simulink model "SixDOF_v2_1c"  (R2019b)
settings: Solver=ode4  StartTime=0  StopTime=200  FixedStep=0.01  RelTol=1e-3
libraries: aerolibconvert2 x11, dspsrcs4 x4, simulink x2
settings Model: SimulationMode=accelerator  Creator=Jared  LastModifiedBy=j90xb
settings SolverCC: AlgebraicLoopSolver=LineSearch
settings DataIOCC: SaveFormat=Array  ReturnWorkspaceOutputs=off
settings DebuggingCC: ArithmeticOperatorsInVariantConditions=warning
settings SFSimCC: SimUseLocalCustomCode=off  CustomCodeUndefinedFunction=UseInterfaceOnly
settings RTWCC: RTWUseLocalCustomCode=off

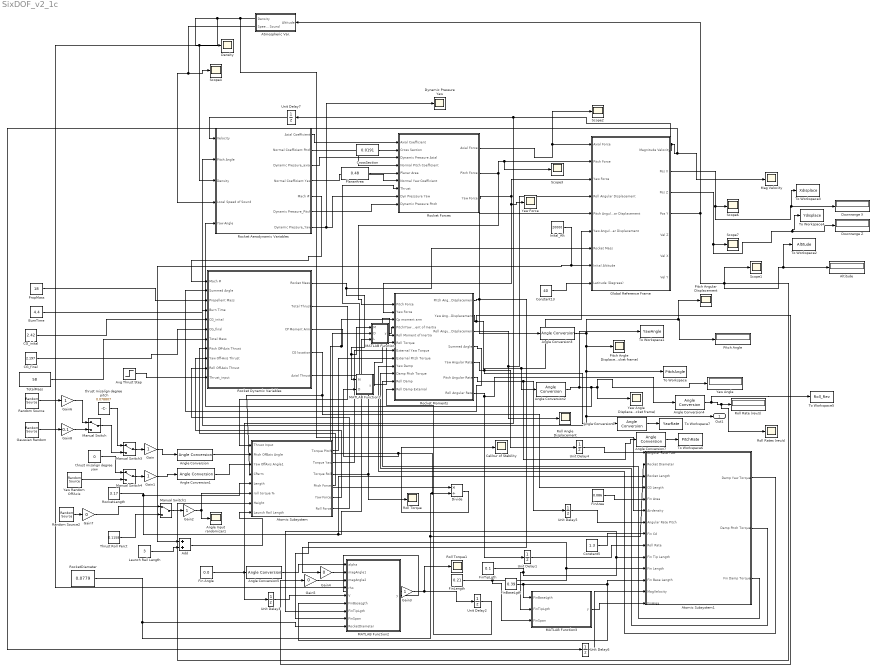
== system SixDOF_v2_1c ==
  Add : Sum
  Altitude : Display
  Angle Conversion : aerolibconvert2/Angle Conversion  IU=deg  OU=rad
  Angle Conversion1 : aerolibconvert2/Angle Conversion  IU=deg  OU=rad
  Angle Conversion{2..3,6..7} (4 alike) : aerolibconvert2/Angle Conversion  IU=rad  OU=deg
  Angle Conversion4 : aerolibconvert2/Angle Conversion  IU=rad  OU=rev
  Angle Conversion5 : aerolibconvert2/Angle Conversion  IU=deg  OU=rad
  Angle Input randomizer1 : Scope
  Atmospheric Var. : Subsystem  TreatAsAtomicUnit=on
  Atomic Subsystem : Subsystem  TreatAsAtomicUnit=on
  Atomic Subsystem1 : Subsystem  TreatAsAtomicUnit=on
  Avg Thrust Step : Step  Time=4.4  Before=8000  After=0
  BurnTime : Constant  Value=4.4
  CG_final : Constant  Value=2.197
  CG_inital : Constant  Value=2.42
  Calibur of Stability : Scope
  Constant13 : Constant  Value=40
  Constant5 : Constant  Value=1.3
  CrossSection : Constant  Value=0.0191
  Density : Scope
  Divide : Product  Inputs=*/
  Downrange X : Display
  Downrange Z : Display
  Dynamic Pressure Yaw : Scope
  Fin Angle : Constant  Value=0.0
  FinArea : Constant  Value=0.086
  FinBaseLgth : Constant  Value=0.39
  FinLength : Constant  Value=0.21
  FinTipLgth : Constant  Value=0.1
  Gain{,1..3,6} (5 alike) : Gain
  Gain4 : Gain  Gain=0
  Gain5 : Gain  Gain=0
  Gain7 : Gain  Gain=0
  Gain8 : Gain  Gain=0.1
  Gaussian Random : dspsrcs4/Random Source  SrcType=Gaussian  NormMethod=Ziggurat  CltLength=12  MinVal=-0.2  MaxVal=0.2  MeanVal=0  VarVal=1  RepMode=Not repeatable  rawSeed=1  IsInherit=off  SampMode=Discrete  SampTime=1  SampFrame=1  DataType=Double  OutComplex=Real  OutputFrames=off
  Global Reference Frame : Subsystem  TreatAsAtomicUnit=on
  Inital_Alt : Constant  Value=20000
  Launch Rail Length : Constant  Value=3
  MATLAB Function : MATLAB Function  TreatAsAtomicUnit=on
  MATLAB Function1 : MATLAB Function  TreatAsAtomicUnit=on
  MATLAB Function2 : MATLAB Function  TreatAsAtomicUnit=on
  MATLAB Function3 : MATLAB Function  TreatAsAtomicUnit=on
  Mag Velocity : Scope
  Manual Switch{,1,3..4} (4 alike) : ManualSwitch
  Pitch Angle : Display
  Pitch Angle Displacement (rocket frame) : Scope
  Pitch Angular Displacement : Scope
  PlanarArea : Constant  Value=0.48
  PropMass : Constant  Value=18
  Random Source : dspsrcs4/Random Source  SrcType=Uniform  NormMethod=Ziggurat  CltLength=12  MinVal=-0.2  MaxVal=0.2  MeanVal=0  VarVal=1  RepMode=Not repeatable  rawSeed=1  IsInherit=off  SampMode=Discrete  SampTime=1000  SampFrame=1  DataType=Double  OutComplex=Real  OutputFrames=off
  Random Source2 : dspsrcs4/Random Source  SrcType=Uniform  NormMethod=Ziggurat  CltLength=12  MinVal=-0.001  MaxVal=0.001  MeanVal=0  VarVal=1  RepMode=Not repeatable  rawSeed=1  IsInherit=off  SampMode=Discrete  SampTime=0.5  SampFrame=1  DataType=Double  OutComplex=Real  OutputFrames=off
  Rocket Aerodynamic Variables : Subsystem  TreatAsAtomicUnit=on
  "Rocket Dynamic Variables " : Subsystem  TreatAsAtomicUnit=on
  Rocket Forces : Subsystem  TreatAsAtomicUnit=on
  Rocket Moments : Subsystem  TreatAsAtomicUnit=on
  RocketDiameter : Constant  Value=0.0779
  RocketLength : Constant  Value=3.17
  Roll Angle Displacement : Scope
  Roll Rate (rev/s) : Display
  Roll Rates (rev/s) : Scope
  Roll Torque : Scope
  Roll Torque1 : Scope
  Scope{1..4,6..7} (6 alike) : Scope
  Thrust Roll Perct : Constant  Value=0.1158
  To Workspace : ToWorkspace  VariableName=PitchAngle  SampleTime=-1
  To Workspace1 : ToWorkspace  VariableName=YawAngle  SampleTime=-1
  To Workspace2 : ToWorkspace  VariableName=Altitude  SampleTime=-1
  To Workspace3 : ToWorkspace  VariableName=Xdisplace  SampleTime=-1
  To Workspace4 : ToWorkspace  VariableName=Ydisplace  SampleTime=-1
  To Workspace5 : ToWorkspace  VariableName=Roll_Rev  SampleTime=-1
  To Workspace6 : ToWorkspace  VariableName=PitchRate  SampleTime=-1
  To Workspace7 : ToWorkspace  VariableName=YawRate  SampleTime=-1
  TotalMass : Constant  Value=58
  Unit Delay{1..7} (7 alike) : UnitDelay  SampleTime=-1  HasFrameUpgradeWarning=on
  Yaw Angle : Display
  Yaw Angle Displacement (rocket frame) : Scope
  Yaw Force : Scope
  Yaw Random OffAxis : dspsrcs4/Random Source  SrcType=Uniform  NormMethod=Ziggurat  CltLength=12  MinVal=-0.02  MaxVal=0.02  MeanVal=0  VarVal=1  RepMode=Not repeatable  rawSeed=1  IsInherit=off  SampMode=Discrete  SampTime=1000  SampFrame=1  DataType=Double  OutComplex=Real  OutputFrames=off
  thrust misalign degree pitch : Constant  Value=0.078807
  thrust misalign degree yaw : Constant  Value=0
  Out1 : Outport  VectorParamsAs1DForOutWhenUnconnected=off
  wires:
  Rocket Forces/1(Axial Force) -> Scope2/1, Global Reference Frame/1(Axial Force)
  Rocket Moments/1(Pitch Angular Displacement) -> Gain4/1, Angle Conversion3/1, Global Reference Frame/5(Pitch Angular Displacement)
  Global Reference Frame/1(Magnitude Velocity) -> Unit Delay3/1, Unit Delay7/1, Unit Delay6/1, Mag Velocity/1
  Global Reference Frame/4(Pos Y) -> Atmospheric Var./1(Altitude), Atomic Subsystem/7(Height), To Workspace2/1, Altitude/1, Scope1/1
  "Rocket Dynamic Variables "/3(CP Moment Arm) -> Divide/1, Rocket Moments/3(Cp moment arm)
  PropMass/1 -> "Rocket Dynamic Variables "/3(Propellent Mass)
  BurnTime/1 -> "Rocket Dynamic Variables "/4(Burn Time)
  CG_inital/1 -> "Rocket Dynamic Variables "/5(CG_inital)
  CG_final/1 -> "Rocket Dynamic Variables "/6(CG_final)
  TotalMass/1 -> "Rocket Dynamic Variables "/7(Total Mass)
  MATLAB Function/1(y) -> Rocket Moments/4(Pitch/Yaw Moment of Inertia)
  CrossSection/1 -> Rocket Forces/2(Cross Section)
  PlanarArea/1 -> Rocket Forces/5(Planar Area)
  Inital_Alt/1 -> Add/1, Global Reference Frame/8(Inital Altitude)
  Atmospheric Var./2(Speed of Sound) -> Scope4/1, Rocket Aerodynamic Variables/4(Local Speed of Sound)
  Global Reference Frame/2(Pos X) -> To Workspace3/1, Downrange X/1, Scope6/1
  Global Reference Frame/3(Pos Z) -> To Workspace4/1, Downrange Z/1, Scope7/1
  Atomic Subsystem/1(Torque Pitch) -> Rocket Moments/8(External Pitch Torque)
  Atomic Subsystem/2(Torque Yaw) -> Rocket Moments/7(External Yaw Torque)
  Angle Conversion/1 -> Atomic Subsystem/2(Pitch OffAxis Angle)
  Angle Conversion1/1 -> Atomic Subsystem/3(Yaw OffAxis Angle1)
  RocketLength/1 -> Atomic Subsystem1/3(Rocket Length), MATLAB Function/3(L), Atomic Subsystem/5(Length)
  Divide/1 -> Calibur of Stability/1
  Atomic Subsystem/3(Torque Roll) -> Roll Torque/1, Rocket Moments/6(Roll Torque)
  MATLAB Function1/1(y) -> Rocket Moments/5(Roll Moment of Inertia)
  Gain/1 -> Angle Conversion/1
  Gain1/1 -> Angle Conversion1/1
  Gain2/1 -> Atomic Subsystem/6(roll torque %), Angle Input randomizer1/1
  RocketDiameter/1 -> MATLAB Function2/9(RocketDiameter), Atomic Subsystem1/2(Rocket Diameter), MATLAB Function1/2(D), MATLAB Function/2(D), Divide/2
  "Rocket Dynamic Variables "/4(CG location) -> Atomic Subsystem1/4(CG Length), Atomic Subsystem/4(CParm)
  "Rocket Dynamic Variables "/1(Rocket Mass) -> MATLAB Function/1(M), MATLAB Function1/1(M), Global Reference Frame/7(Rocket Mass)
  Rocket Forces/3(Yaw Force) -> Rocket Moments/2(Yaw Force), Yaw Force/1, Global Reference Frame/3(Yaw Force)
  Rocket Moments/3(Roll Angular Displacement) -> Roll Angle Displacement/1, Global Reference Frame/4(Roll Angular Displacement)
  "Rocket Dynamic Variables "/5(Axial Thrust) -> Rocket Forces/7(Thrust)
  Rocket Aerodynamic Variables/5(Mach #) -> "Rocket Dynamic Variables "/1("Mach # ")
  Rocket Aerodynamic Variables/1(" Axial Coefficient") -> Rocket Forces/1(Axial Coefficient)
  Rocket Aerodynamic Variables/3(Dynamic Pressure_axial) -> Rocket Forces/3(Dynamic Pressure Axial)
  Rocket Aerodynamic Variables/2(" Normal Coefficient Pitch") -> Rocket Forces/4(Normal Pitch Coefficient)
  Rocket Aerodynamic Variables/4(" Normal Coefficient Yaw") -> Rocket Forces/6(Normal Yaw Coefficient)
  "Rocket Dynamic Variables "/2(Total Thrust) -> Atomic Subsystem/1(Thrust Input)
  Atmospheric Var./1(Density) -> Atomic Subsystem1/6(Airdensity), MATLAB Function2/4(rho), Density/1, Rocket Aerodynamic Variables/3(Density)
  Rocket Moments/4(Summed Angle) -> "Rocket Dynamic Variables "/2(Summed Angle)
  Atomic Subsystem/4(Pitch Force) -> "Rocket Dynamic Variables "/8(Pitch Off-Axis Thrust)
  Atomic Subsystem/5(Yaw Force) -> "Rocket Dynamic Variables "/9(Yaw Off-Axis Thrust)
  Atomic Subsystem/6(Roll Force) -> "Rocket Dynamic Variables "/10(Roll Off-Axis Thrust)
  Rocket Aerodynamic Variables/6(Dynamic Pressure_Pitch) -> Rocket Forces/9(Dynamic Pressure Pitch)
  Rocket Aerodynamic Variables/7(Dynamic Pressure_Yaw) -> Dynamic Pressure Yaw/1, Rocket Forces/8(Dyn Presssure Yaw)
  Unit Delay7/1 -> Rocket Aerodynamic Variables/1(Velocity)
  Rocket Moments/2(Yaw Angular Displacement) -> Gain5/1, Global Reference Frame/6(Yaw Angular Displacement), Angle Conversion2/1
  Rocket Moments/5(Yaw Angular Rate) -> Angle Conversion6/1, Unit Delay4/1
  FinArea/1 -> Atomic Subsystem1/5(Fin Area)
  Atomic Subsystem1/1(Damp Yaw Torque) -> Rocket Moments/9(Yaw Damp)
  Unit Delay4/1 -> Atomic Subsystem1/1(Angular Rate Yaw)
  Angle Conversion2/1 -> To Workspace1/1, Rocket Aerodynamic Variables/5(Yaw Angle), Yaw Angle/1, Yaw Angle Displacement (rocket frame)/1
  Atomic Subsystem1/2(Damp Pitch Torque) -> Rocket Moments/10(Damp Pitch Torque)
  Rocket Moments/6(Pitch Angular Rate) -> Angle Conversion7/1, Unit Delay5/1
  Unit Delay5/1 -> Atomic Subsystem1/7(Angular Rate Pitch)
  Gaussian Random/1 -> Gain8/1
  Random Source/1 -> Gain6/1
  Manual Switch1/1 -> Gain2/1
  Random Source2/1 -> Gain7/1
  Thrust Roll Perct/1 -> Manual Switch1/2
  Constant13/1 -> Global Reference Frame/9(Latitude (Degrees))
  Launch Rail Length/1 -> Add/2
  Add/1 -> Atomic Subsystem/8(Launch Rail Length)
  Angle Conversion3/1 -> Rocket Aerodynamic Variables/2(Pitch Angle), Out1/1, To Workspace/1, Pitch Angle Displacement (rocket frame)/1, Pitch Angle/1, Pitch Angular Displacement/1
  Atomic Subsystem1/3(Fin Damp Torque) -> Rocket Moments/11(Roll Damp)
  Rocket Moments/7(Roll Angular Rate) -> Angle Conversion4/1, Unit Delay1/1
  Constant5/1 -> Atomic Subsystem1/8(Fin Cd)
  FinTipLgth/1 -> MATLAB Function3/2(FinTipLgth), Atomic Subsystem1/10(Fin Tip Length), MATLAB Function2/7(FinTipLgth)
  FinLength/1 -> MATLAB Function3/3(FinSpan), MATLAB Function2/8(FinSpan), Atomic Subsystem1/11(Fin Length)
  FinBaseLgth/1 -> MATLAB Function3/1(FinBaseLgth), MATLAB Function2/6(FinBaseLgth), Atomic Subsystem1/12(Fin Base Length)
  Unit Delay1/1 -> Atomic Subsystem1/9(Roll Rate)
  MATLAB Function2/1(y) -> Gain3/1
  Angle Conversion5/1 -> MATLAB Function2/1(alpha)
  Fin Angle/1 -> Angle Conversion5/1
  Unit Delay2/1 -> Rocket Moments/12(Roll Damp External)
  Unit Delay3/1 -> MATLAB Function2/5(V)
  MATLAB Function3/1(y) -> Atomic Subsystem1/14(FinArea)
  Unit Delay6/1 -> Atomic Subsystem1/13(MagVelocity)
  Angle Conversion4/1 -> To Workspace5/1, Roll Rates (rev/s)/1, Roll Rate (rev/s)/1
  Gain3/1 -> Roll Torque1/1, Unit Delay2/1
  Rocket Forces/2(Pitch Force) -> Rocket Moments/1(Pitch Force), Scope3/1, Global Reference Frame/2(Pitch Force)
  Angle Conversion7/1 -> To Workspace6/1
  Angle Conversion6/1 -> To Workspace7/1
  Gain4/1 -> MATLAB Function2/2(magAngle1)
  Gain5/1 -> MATLAB Function2/3(magAngle2)
  Gain7/1 -> Manual Switch1/1
  Gain6/1 -> Manual Switch/1
  Gain8/1 -> Manual Switch/2
  Manual Switch3/1 -> Gain/1
  Manual Switch4/1 -> Gain1/1
  Yaw Random OffAxis/1 -> Manual Switch4/2
  Manual Switch/1 -> Manual Switch3/2
  thrust misalign degree pitch/1 -> Manual Switch3/1
  thrust misalign degree yaw/1 -> Manual Switch4/1
  Avg Thrust Step/1 -> "Rocket Dynamic Variables "/11(Thrust_input)

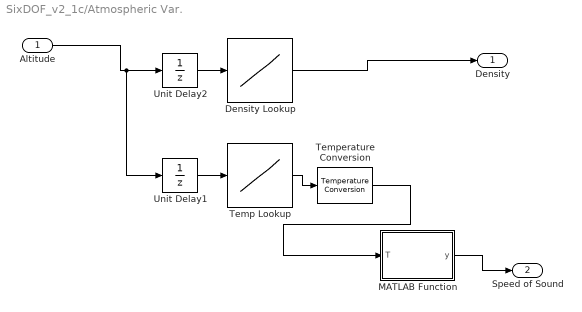
== system SixDOF_v2_1c/Atmospheric Var. ==
  Altitude : Inport
  Density Lookup : Lookup_n-D  NumberOfTableDimensions=1  BreakpointsForDimension1=[0,1000,2000,3000,4000,5000,6000,7000,8000,9000,10000,15000,20000,25000,30000,40000,50000,60000,70000,80000,120000]  Table=[1.347,1.225,1.112,1.007,0.9093,0.8194,0.7364,0.6601,0.59,0.4671,0.4135,0.1948,0.0889,0.04,0.0184,0.003996,0.001027,0.0003097,8.283e-05,0.00001846,1e-07]  InterpMethod=Cubic spline  InternalRulePriority=Speed  RndMeth=Simplest  InputSameDT=on
  MATLAB Function : MATLAB Function  TreatAsAtomicUnit=on
  Temp Lookup : Lookup_n-D  NumberOfTableDimensions=1  BreakpointsForDimension1=[0,1000,2000,3000,4000,5000,6000,7000,8000,9000,10000,15000,20000,25000,30000,40000,50000,60000,70000,80000,120000]  Table=[21.50,8.5,2,-4.49,-10.98,-17.47,-23.96,-30.45,-36.95,-43.42,-49.90,-56.50,-56.50,-51.60,-46.64,-22.80,-2.5,-26.13,-53.57,-74.51,-80]  InternalRulePriority=Speed  RndMeth=Simplest  InputSameDT=on
  Temperature Conversion : aerolibconvert2/Temperature Conversion  IU=C  OU=K
      settings: SourceProductName=Aerospace Blockset  SourceProductBaseCode=AE
  Unit Delay1 : UnitDelay  SampleTime=-1  HasFrameUpgradeWarning=on
  Unit Delay2 : UnitDelay  SampleTime=-1  HasFrameUpgradeWarning=on
  Density : Outport  VectorParamsAs1DForOutWhenUnconnected=off
  Speed of Sound : Outport  Port=2  VectorParamsAs1DForOutWhenUnconnected=off
  wires:
  Altitude/1 -> Unit Delay2/1, Unit Delay1/1
  Temp Lookup/1 -> Temperature Conversion/1
  MATLAB Function/1(y) -> Speed of Sound/1
  Temperature Conversion/1 -> MATLAB Function/1(T)
  Density Lookup/1 -> Density/1
  Unit Delay1/1 -> Temp Lookup/1
  Unit Delay2/1 -> Density Lookup/1

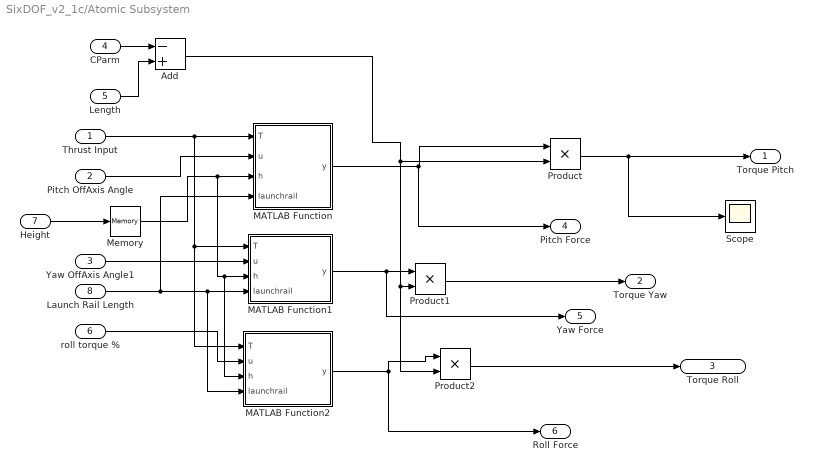
== system SixDOF_v2_1c/Atomic Subsystem ==
  Thrust Input : Inport
  Pitch OffAxis Angle : Inport  Port=2
  Yaw OffAxis Angle1 : Inport  Port=3
  CParm : Inport  Port=4
  Length : Inport  Port=5
  roll torque % : Inport  Port=6
  Height : Inport  Port=7
  Launch Rail Length : Inport  Port=8
  Add : Sum  Inputs=-+
  MATLAB Function : MATLAB Function  TreatAsAtomicUnit=on
  MATLAB Function1 : MATLAB Function  TreatAsAtomicUnit=on
  MATLAB Function2 : MATLAB Function  TreatAsAtomicUnit=on
  Memory : Memory
  Product : Product
  Product1 : Product
  Product2 : Product
  Scope : Scope
  Torque Pitch : Outport  VectorParamsAs1DForOutWhenUnconnected=off
  Torque Yaw : Outport  Port=2  VectorParamsAs1DForOutWhenUnconnected=off
  Torque Roll : Outport  Port=3  VectorParamsAs1DForOutWhenUnconnected=off
  Pitch Force : Outport  Port=4  VectorParamsAs1DForOutWhenUnconnected=off
  Yaw Force : Outport  Port=5  VectorParamsAs1DForOutWhenUnconnected=off
  Roll Force : Outport  Port=6  VectorParamsAs1DForOutWhenUnconnected=off
  wires:
  CParm/1 -> Add/1
  Length/1 -> Add/2
  MATLAB Function1/1(y) -> Yaw Force/1, Product1/1
  Product1/1 -> Torque Yaw/1
  Product2/1 -> Torque Roll/1
  MATLAB Function2/1(y) -> Product2/1, Roll Force/1
  Product/1 -> Torque Pitch/1, Scope/1
  MATLAB Function/1(y) -> Pitch Force/1, Product/1
  Add/1 -> Product2/2, Product1/2, Product/2
  Thrust Input/1 -> MATLAB Function2/1(T), MATLAB Function1/1(T), MATLAB Function/1(T)
  Pitch OffAxis Angle/1 -> MATLAB Function/2(u)
  roll torque %/1 -> MATLAB Function2/2(u)
  Yaw OffAxis Angle1/1 -> MATLAB Function1/2(u)
  Height/1 -> Memory/1
  Launch Rail Length/1 -> MATLAB Function/4(launchrail), MATLAB Function2/4(launchrail), MATLAB Function1/4(launchrail)
  Memory/1 -> MATLAB Function2/3(h), MATLAB Function1/3(h), MATLAB Function/3(h)

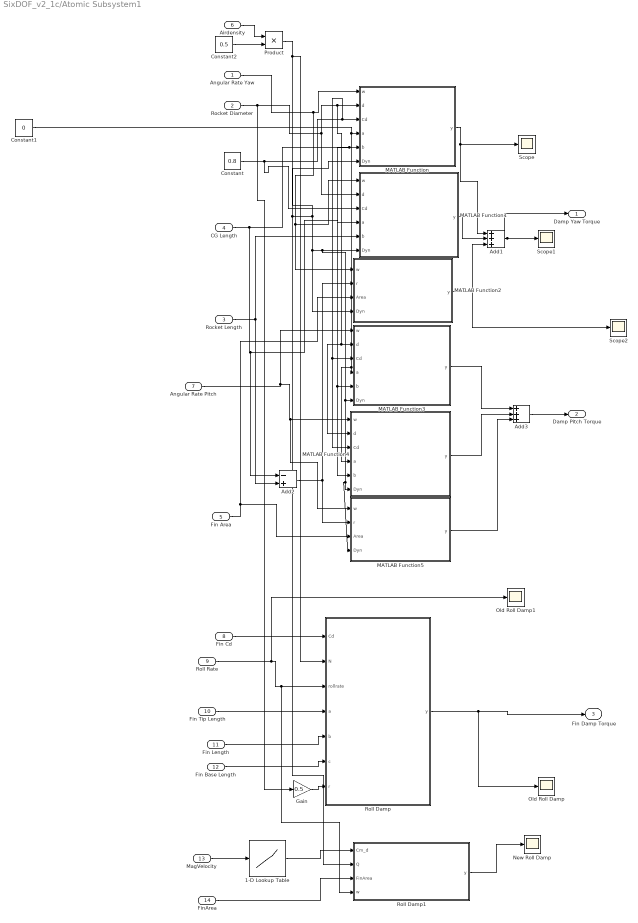
== system SixDOF_v2_1c/Atomic Subsystem1 ==
  Angular Rate Yaw : Inport
  Rocket Diameter : Inport  Port=2
  Rocket Length : Inport  Port=3
  CG Length : Inport  Port=4
  Fin Area : Inport  Port=5
  Airdensity : Inport  Port=6
  Angular Rate Pitch : Inport  Port=7
  Fin Cd : Inport  Port=8
  Roll Rate : Inport  Port=9
  Fin Tip Length : Inport  Port=10
  Fin Length : Inport  Port=11
  Fin Base Length : Inport  Port=12
  MagVelocity : Inport  Port=13
  FinArea : Inport  Port=14
  1-D Lookup Table : Lookup_n-D  NumberOfTableDimensions=1  BreakpointsForDimension1=[0,0.1,0.5,1,2,3,4,5]  Table=[2,0.65,0.61,0.75,0.25,0.2,0.18,0.17]  InternalRulePriority=Speed  RndMeth=Simplest  InputSameDT=on
  Add1 : Sum  Inputs=+++
  Add2 : Sum  Inputs=-+
  Add3 : Sum  Inputs=+++
  Constant : Constant  Value=0.8
  Constant1 : Constant  Value=0
  Constant2 : Constant  Value=0.5
  Gain : Gain  Gain=0.5
  MATLAB Function : MATLAB Function  TreatAsAtomicUnit=on
  MATLAB Function1 : MATLAB Function  TreatAsAtomicUnit=on
  MATLAB Function2 : MATLAB Function  TreatAsAtomicUnit=on
  MATLAB Function3 : MATLAB Function  TreatAsAtomicUnit=on
  MATLAB Function4 : MATLAB Function  TreatAsAtomicUnit=on
  MATLAB Function5 : MATLAB Function  TreatAsAtomicUnit=on
  New Roll Damp : Scope
  Old Roll Damp : Scope
  Old Roll Damp1 : Scope
  Product : Product
  Roll Damp : MATLAB Function  TreatAsAtomicUnit=on
  Roll Damp1 : MATLAB Function  TreatAsAtomicUnit=on
  Scope : Scope
  Scope1 : Scope
  Scope2 : Scope
  Damp Yaw Torque : Outport  VectorParamsAs1DForOutWhenUnconnected=off
  Damp Pitch Torque : Outport  Port=2  VectorParamsAs1DForOutWhenUnconnected=off
  Fin Damp Torque : Outport  Port=3  VectorParamsAs1DForOutWhenUnconnected=off
  wires:
  Angular Rate Yaw/1 -> MATLAB Function2/1(w), MATLAB Function1/1(w), MATLAB Function/1(w)
  Constant/1 -> MATLAB Function4/3(Cd), MATLAB Function3/3(Cd), MATLAB Function/3(Cd), MATLAB Function1/3(Cd)
  Constant1/1 -> MATLAB Function4/4(a), MATLAB Function3/4(a), MATLAB Function/4(a)
  MATLAB Function/1(y) -> Add1/1, Scope/1
  CG Length/1 -> Add2/1, MATLAB Function1/4(a), MATLAB Function4/5(b), MATLAB Function3/5(b), MATLAB Function/5(b)
  Rocket Length/1 -> Add2/2, MATLAB Function1/5(b)
  MATLAB Function1/1(y) -> Add1/2
  Add1/1 -> Damp Yaw Torque/1, Scope1/1
  Airdensity/1 -> Product/1
  Constant2/1 -> Product/2
  Product/1 -> Roll Damp/2(N), Roll Damp1/2(Q), MATLAB Function2/4(Dyn), MATLAB Function5/4(Dyn), MATLAB Function4/6(Dyn), MATLAB Function3/6(Dyn), MATLAB Function1/6(Dyn), MATLAB Function/6(Dyn)
  Add2/1 -> MATLAB Function2/2(r), MATLAB Function5/2(r)
  Fin Area/1 -> MATLAB Function5/3(Area), MATLAB Function2/3(Area)
  MATLAB Function2/1(y) -> Add1/3, Scope2/1
  Angular Rate Pitch/1 -> MATLAB Function5/1(w), MATLAB Function4/1(w), MATLAB Function3/1(w)
  MATLAB Function3/1(y) -> Add3/1
  MATLAB Function4/1(y) -> Add3/2
  MATLAB Function5/1(y) -> Add3/3
  Add3/1 -> Damp Pitch Torque/1
  Roll Rate/1 -> Old Roll Damp1/1, Roll Damp1/4(w), Roll Damp/3(rollrate)
  Fin Tip Length/1 -> Roll Damp/4(a)
  Gain/1 -> Roll Damp/7(r)
  Fin Base Length/1 -> Roll Damp/6(c)
  Fin Cd/1 -> Roll Damp/1(Cd)
  Fin Length/1 -> Roll Damp/5(b)
  Rocket Diameter/1 -> Gain/1, MATLAB Function1/2(d), MATLAB Function4/2(d), MATLAB Function3/2(d), MATLAB Function/2(d)
  MagVelocity/1 -> 1-D Lookup Table/1
  1-D Lookup Table/1 -> Roll Damp1/1(Cm_d)
  FinArea/1 -> Roll Damp1/3(FinArea)
  Roll Damp1/1(y) -> New Roll Damp/1
  Roll Damp/1(y) -> Old Roll Damp/1, Fin Damp Torque/1

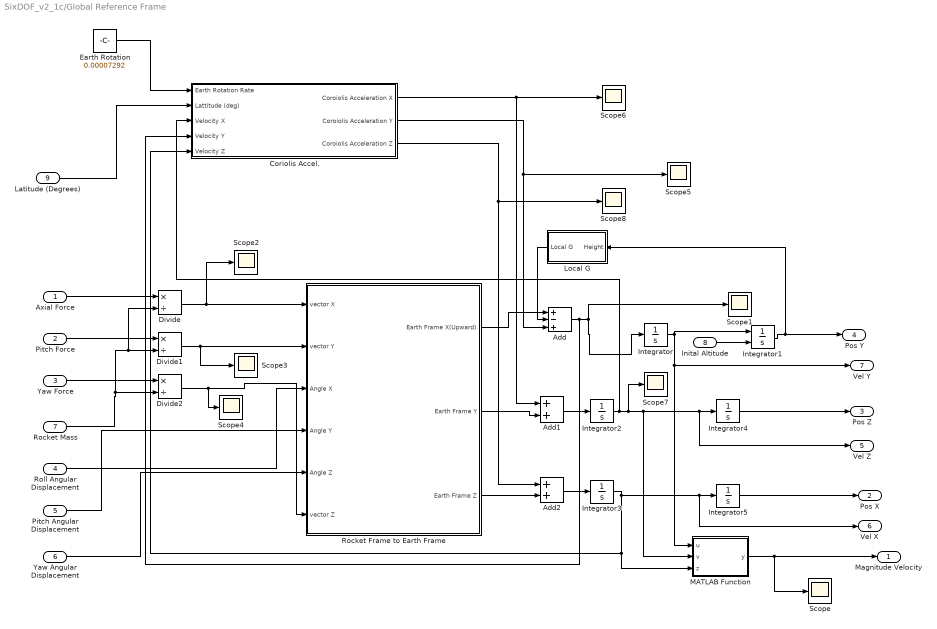
== system SixDOF_v2_1c/Global Reference Frame ==
  Axial Force : Inport
  Pitch Force : Inport  Port=2
  Yaw Force : Inport  Port=3
  Roll Angular Displacement : Inport  Port=4
  Pitch Angular Displacement : Inport  Port=5
  Yaw Angular Displacement : Inport  Port=6
  Rocket Mass : Inport  Port=7
  Inital Altitude : Inport  Port=8
  Latitude (Degrees) : Inport  Port=9
  Add : Sum  Inputs=+-+
  Add1 : Sum
  Add2 : Sum
  Coriolis Accel. : Subsystem
  Divide : Product  Inputs=*/
  Divide1 : Product  Inputs=*/
  Divide2 : Product  Inputs=*/
  Earth Rotation : Constant  Value=0.00007292
  Integrator{,2..5} (5 alike) : Integrator
  Integrator1 : Integrator  InitialConditionSource=external
  Local G : Subsystem
  MATLAB Function : MATLAB Function  TreatAsAtomicUnit=on
  Rocket Frame to Earth Frame : Subsystem
  Scope{,1..8} (9 alike) : Scope
  Magnitude Velocity : Outport  VectorParamsAs1DForOutWhenUnconnected=off
  Pos X : Outport  Port=2  VectorParamsAs1DForOutWhenUnconnected=off
  Pos Z : Outport  Port=3  VectorParamsAs1DForOutWhenUnconnected=off
  Pos Y : Outport  Port=4  VectorParamsAs1DForOutWhenUnconnected=off
  Vel Z : Outport  Port=5  VectorParamsAs1DForOutWhenUnconnected=off
  Vel X : Outport  Port=6  VectorParamsAs1DForOutWhenUnconnected=off
  "Vel Y " : Outport  Port=7  VectorParamsAs1DForOutWhenUnconnected=off
  wires:
  Divide/1 -> Rocket Frame to Earth Frame/1(vector X), Scope2/1
  Divide1/1 -> Rocket Frame to Earth Frame/2(vector Y), Scope3/1
  Divide2/1 -> Rocket Frame to Earth Frame/6(vector Z), Scope4/1
  Local G/1(Local G) -> Add/2
  Add/1 -> Coriolis Accel./4(Velocity Y), Integrator/1, Scope1/1
  Integrator3/1 -> Coriolis Accel./5(Velocity Z), MATLAB Function/3(z), Vel X/1, Integrator5/1
  Integrator5/1 -> Pos X/1
  Integrator4/1 -> Pos Z/1
  Inital Altitude/1 -> Integrator1/2
  MATLAB Function/1(y) -> Magnitude Velocity/1, Scope/1
  Integrator1/1 -> Local G/1(Height), Pos Y/1
  Integrator2/1 -> Coriolis Accel./3(Velocity X), Scope7/1, MATLAB Function/2(v), Vel Z/1, Integrator4/1
  Integrator/1 -> "Vel Y "/1, MATLAB Function/1(u), Integrator1/1
  Yaw Angular Displacement/1 -> Rocket Frame to Earth Frame/5(Angle Z)
  Yaw Force/1 -> Divide2/1
  Pitch Force/1 -> Divide1/1
  Rocket Frame to Earth Frame/1(Earth Frame X(Upward)) -> Add/1
  Axial Force/1 -> Divide/1
  Rocket Mass/1 -> Divide/2, Divide1/2, Divide2/2
  Roll Angular Displacement/1 -> Rocket Frame to Earth Frame/3(Angle X)
  Pitch Angular Displacement/1 -> Rocket Frame to Earth Frame/4(Angle Y)
  Earth Rotation/1 -> Coriolis Accel./1(Earth Rotation Rate)
  Latitude (Degrees)/1 -> Coriolis Accel./2(Lattitude (deg))
  Add1/1 -> Integrator2/1
  Rocket Frame to Earth Frame/2(Earth Frame Y) -> Add1/2
  Coriolis Accel./2(Coroiolis Acceleration Y) -> Scope5/1, Add/3
  Coriolis Accel./3(Coroiolis Acceleration Z) -> Scope8/1, Add2/1
  Coriolis Accel./1(Coroiolis Acceleration X) -> Scope6/1, Add1/1
  Add2/1 -> Integrator3/1
  Rocket Frame to Earth Frame/3(Earth Frame Z) -> Add2/2

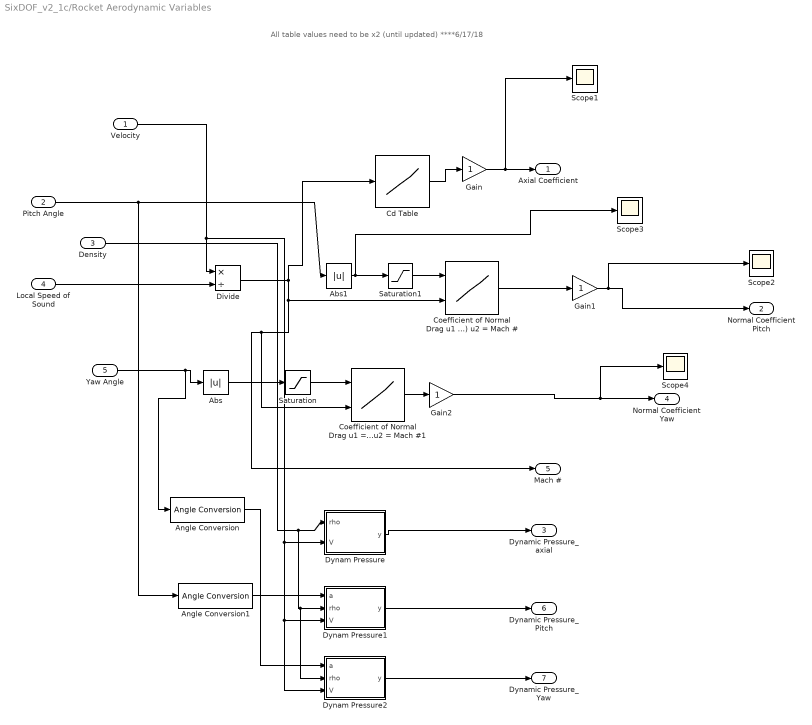
== system SixDOF_v2_1c/Rocket Aerodynamic Variables ==
  note: All table values need to be x2 (until updated) ****6/17/18
  Velocity : Inport
  Pitch Angle : Inport  Port=2
  Density : Inport  Port=3
  Local Speed of Sound : Inport  Port=4
  Yaw Angle : Inport  Port=5
  Abs : Abs
  Abs1 : Abs
  Angle Conversion : aerolibconvert2/Angle Conversion  IU=deg  OU=rad
  Angle Conversion1 : aerolibconvert2/Angle Conversion  IU=deg  OU=rad
  Cd Table : Lookup_n-D  NumberOfTableDimensions=1  BreakpointsForDimension1=[0,0.05,0.1,0.6,0.9,1.1,1.2,2,3,4,5]  Table=[0.48,0.4,0.42,0.4,0.44,0.54,0.52,0.36,0.24,0.18,0.14]  InternalRulePriority=Speed  RndMeth=Simplest  InputSameDT=on
  Coefficient of Normal Drag u1 = AOA (Degrees) u2 = Mach # : Lookup_n-D  BreakpointsForDimension1=[0,2,4,6,8,10,12,14,15]  BreakpointsForDimension2=[0,0.5,1.1,2,5]  Table=reshape([1e-06,0.6,1.25,1.9,2.5,3.2,3.6,4.2,4.5,1e-06,0.6,1.25,1.9,2.5,3.2,3.6,4.2,4.5,1e-06,0.8,1.6,2.5,3.4,4.2,5,5.8,6.2,1e-06,0.7,1.4,2,2.5,3.2,4,5.6,6.2,1e-06,0.25,0.8,1.4,2,2.6,3.2,3.9,3.3],9,5)  ExtrapMethod=Clip  UseLastTableValue=on  InternalRulePriority=Speed  RndMeth=Simplest  InputSameDT=on
  Coefficient of Normal Drag u1 = AOA (Degrees) u2 = Mach #1 : Lookup_n-D  BreakpointsForDimension1=[0,2,4,6,8,10,12,14,15]  BreakpointsForDimension2=[0,0.5,1.1,2,5]  Table=reshape([1e-06,0.6,1.25,1.9,2.5,3.2,3.6,4.2,4.5,1e-06,0.6,1.25,1.9,2.5,3.2,3.6,4.2,4.5,1e-06,0.8,1.6,2.5,3.4,4.2,5,5.8,6.2,1e-06,0.7,1.4,2,2.5,3.2,4,5.6,6.2,1e-06,0.25,0.8,1.4,2,2.6,3.2,3.9,3.3],9,5)  ExtrapMethod=Clip  UseLastTableValue=on  InternalRulePriority=Speed  RndMeth=Simplest  InputSameDT=on
  Divide : Product  Inputs=*/
  Dynam Pressure : MATLAB Function  TreatAsAtomicUnit=on
  Dynam Pressure1 : MATLAB Function  TreatAsAtomicUnit=on
  Dynam Pressure2 : MATLAB Function  TreatAsAtomicUnit=on
  Gain : Gain
  Gain1 : Gain
  Gain2 : Gain
  Saturation : Saturate  UpperLimit=90  LowerLimit=0
  Saturation1 : Saturate  UpperLimit=90  LowerLimit=0
  Scope{1..4} (4 alike) : Scope
  " Axial Coefficient" : Outport  VectorParamsAs1DForOutWhenUnconnected=off
  " Normal Coefficient Pitch" : Outport  Port=2  VectorParamsAs1DForOutWhenUnconnected=off
  Dynamic Pressure_axial : Outport  Port=3  VectorParamsAs1DForOutWhenUnconnected=off
  " Normal Coefficient Yaw" : Outport  Port=4  VectorParamsAs1DForOutWhenUnconnected=off
  Mach # : Outport  Port=5  VectorParamsAs1DForOutWhenUnconnected=off
  Dynamic Pressure_Pitch : Outport  Port=6  VectorParamsAs1DForOutWhenUnconnected=off
  Dynamic Pressure_Yaw : Outport  Port=7  VectorParamsAs1DForOutWhenUnconnected=off
  wires:
  Local Speed of Sound/1 -> Divide/2
  Divide/1 -> Cd Table/1, Coefficient of Normal Drag u1 = AOA (Degrees) u2 = Mach #/2, Coefficient of Normal Drag u1 = AOA (Degrees) u2 = Mach #1/2, Mach #/1
  Coefficient of Normal Drag u1 = AOA (Degrees) u2 = Mach #/1 -> Gain1/1
  Coefficient of Normal Drag u1 = AOA (Degrees) u2 = Mach #1/1 -> Gain2/1
  Cd Table/1 -> Gain/1
  Dynam Pressure/1(y) -> Dynamic Pressure_axial/1
  Gain/1 -> Scope1/1, " Axial Coefficient"/1
  Density/1 -> Dynam Pressure2/2(rho), Dynam Pressure1/2(rho), Dynam Pressure/1(rho)
  Pitch Angle/1 -> Abs1/1, Angle Conversion1/1
  Velocity/1 -> Dynam Pressure2/3(V), Dynam Pressure1/3(V), Dynam Pressure/2(V), Divide/1
  Dynam Pressure1/1(y) -> Dynamic Pressure_Pitch/1
  Dynam Pressure2/1(y) -> Dynamic Pressure_Yaw/1
  Angle Conversion1/1 -> Dynam Pressure1/1(a)
  Angle Conversion/1 -> Dynam Pressure2/1(a)
  Abs/1 -> Saturation/1
  Abs1/1 -> Scope3/1, Saturation1/1
  Yaw Angle/1 -> Angle Conversion/1, Abs/1
  Gain2/1 -> Scope4/1, " Normal Coefficient Yaw"/1
  Gain1/1 -> Scope2/1, " Normal Coefficient Pitch"/1
  Saturation/1 -> Coefficient of Normal Drag u1 = AOA (Degrees) u2 = Mach #1/1
  Saturation1/1 -> Coefficient of Normal Drag u1 = AOA (Degrees) u2 = Mach #/1

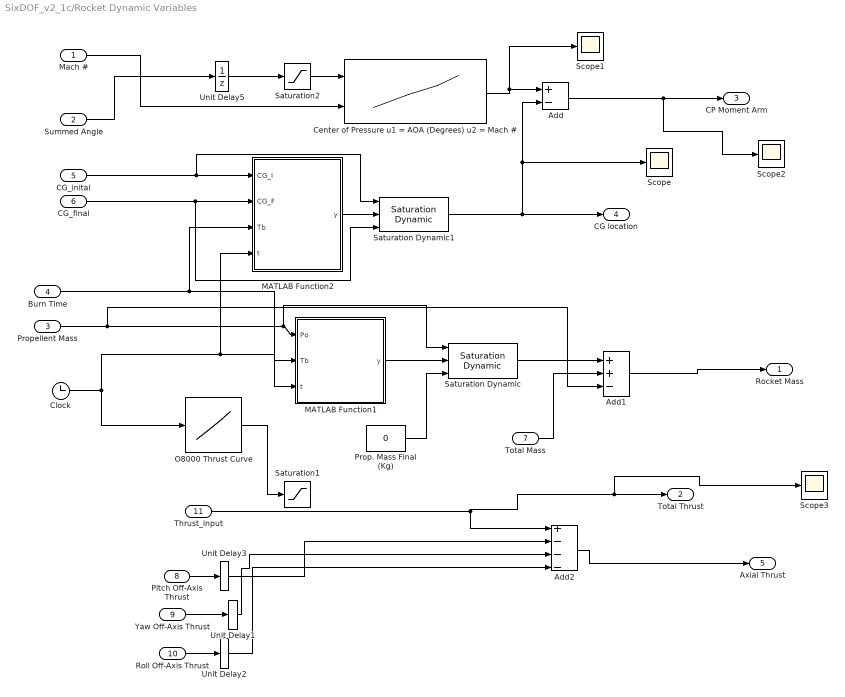
== system SixDOF_v2_1c/Rocket Dynamic Variables  ==
  "Mach # " : Inport
  Summed Angle : Inport  Port=2
  Propellent Mass : Inport  Port=3
  Burn Time : Inport  Port=4
  CG_inital : Inport  Port=5
  CG_final : Inport  Port=6
  Total Mass : Inport  Port=7
  Pitch Off-Axis Thrust : Inport  Port=8
  Yaw Off-Axis Thrust : Inport  Port=9
  Roll Off-Axis Thrust : Inport  Port=10
  Thrust_input : Inport  Port=11
  Add : Sum  Inputs=+-
  Add1 : Sum  Inputs=++-
  Add2 : Sum  Inputs=+---
  Center of Pressure u1 = AOA (Degrees) u2 = Mach # : Lookup_n-D  BreakpointsForDimension1=[0,2,4]  BreakpointsForDimension2=[0,0.9,0.95,1.1,2,3,4,5]  Table=reshape([2.807,2.807,2.807,2.807,2.807,2.807,2.89,2.844,2.807,3,2.89,2.84,2.844,2.769,2.718,2.641,2.616,2.64,2.489,2.47,2.46,2.4,2.36,2.34],3,8)  InterpMethod=Cubic spline  ExtrapMethod=Clip  InternalRulePriority=Speed  RndMeth=Simplest  InputSameDT=on
  Clock : Clock
  MATLAB Function1 : MATLAB Function  TreatAsAtomicUnit=on
  MATLAB Function2 : MATLAB Function  TreatAsAtomicUnit=on
  O8000 Thrust Curve : Lookup_n-D  NumberOfTableDimensions=1  BreakpointsForDimension1=[0,0.056,0.075,0.099,0.124,0.199,0.304,0.491,0.547,0.602,0.671,0.789,0.913,1.019,1.248,1.547,1.901,2.161,2.441,2.714,2.963,3.286,3.59,3.851,4.075,4.28,4.484,4.652,4.77,4.851,4.913,4.969,4.994,5.13,5.161,5.193,5.261]  Table=[0,9389,8412,8106,7740,7938,8183,8519,8595,8488,8396,8335,8320,8381,8427,8519,8549,8549,8503,8412,8290,8122,7984,7832,7709,7587,7511,7465,7435,7389,7297,7267,7145,1053,305,137,0]  InternalRulePriority=Speed  RndMeth=Simplest  InputSameDT=on
  Prop. Mass Final (Kg) : Constant  Value=0
  Saturation Dynamic : simulink/Discontinuities/Saturation Dynamic  OutMin=[]  OutMax=[]  OutDataTypeStr=Inherit: Same as second input  OutDataType=fixdt(1, 16)  OutScaling=2^-10  DoSatur=off
  Saturation Dynamic1 : simulink/Discontinuities/Saturation Dynamic  OutMin=[]  OutMax=[]  OutDataTypeStr=Inherit: Same as second input  OutDataType=fixdt(1, 16)  OutScaling=2^-10  DoSatur=off
  Saturation1 : Saturate  UpperLimit=10000  LowerLimit=0
  Saturation2 : Saturate  UpperLimit=90  LowerLimit=0
  Scope{,1..3} (4 alike) : Scope
  Unit Delay{1..3,5} (4 alike) : UnitDelay  SampleTime=-1  HasFrameUpgradeWarning=on
  Rocket Mass : Outport  VectorParamsAs1DForOutWhenUnconnected=off
  Total Thrust : Outport  Port=2  VectorParamsAs1DForOutWhenUnconnected=off
  CP Moment Arm : Outport  Port=3  VectorParamsAs1DForOutWhenUnconnected=off
  CG location : Outport  Port=4  VectorParamsAs1DForOutWhenUnconnected=off
  Axial Thrust : Outport  Port=5  VectorParamsAs1DForOutWhenUnconnected=off
  wires:
  O8000 Thrust Curve/1 -> Saturation1/1
  MATLAB Function1/1(y) -> Saturation Dynamic/2
  Prop. Mass Final (Kg)/1 -> Saturation Dynamic/3
  Propellent Mass/1 -> Add1/3, Saturation Dynamic/1, MATLAB Function1/1(Po)
  Burn Time/1 -> MATLAB Function2/3(Tb), MATLAB Function1/2(Tb)
  Summed Angle/1 -> Unit Delay5/1
  CG_inital/1 -> Saturation Dynamic1/1, MATLAB Function2/1(CG_I)
  CG_final/1 -> Saturation Dynamic1/3, MATLAB Function2/2(CG_F)
  MATLAB Function2/1(y) -> Saturation Dynamic1/2
  Saturation Dynamic/1 -> Add1/1
  Total Mass/1 -> Add1/2
  Yaw Off-Axis Thrust/1 -> Unit Delay1/1
  Roll Off-Axis Thrust/1 -> Unit Delay2/1
  Center of Pressure u1 = AOA (Degrees) u2 = Mach #/1 -> Scope1/1, Add/1
  Add1/1 -> Rocket Mass/1
  Clock/1 -> O8000 Thrust Curve/1, MATLAB Function2/4(t), MATLAB Function1/3(t)
  Saturation Dynamic1/1 -> CG location/1, Scope/1, Add/2
  Pitch Off-Axis Thrust/1 -> Unit Delay3/1
  Unit Delay1/1 -> Add2/3
  Unit Delay2/1 -> Add2/4
  Add2/1 -> Axial Thrust/1
  Unit Delay3/1 -> Add2/2
  Unit Delay5/1 -> Saturation2/1
  "Mach # "/1 -> Center of Pressure u1 = AOA (Degrees) u2 = Mach #/2
  Add/1 -> Scope2/1, CP Moment Arm/1
  Saturation2/1 -> Center of Pressure u1 = AOA (Degrees) u2 = Mach #/1
  Thrust_input/1 -> Scope3/1, Total Thrust/1, Add2/1

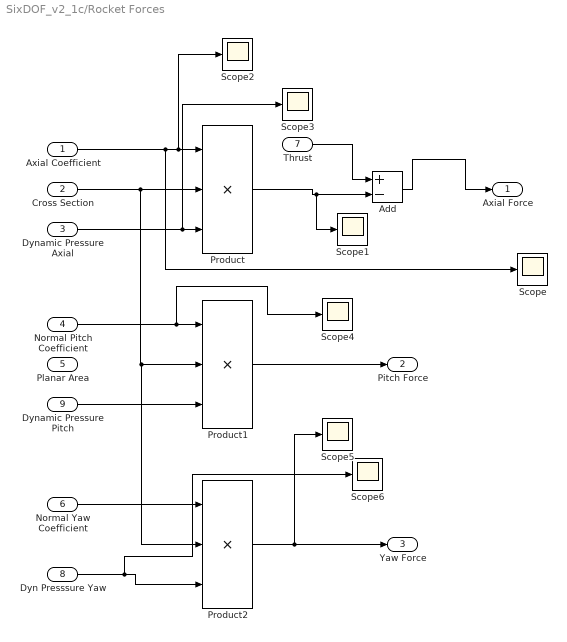
== system SixDOF_v2_1c/Rocket Forces ==
  Axial Coefficient : Inport
  Cross Section : Inport  Port=2
  Dynamic Pressure Axial : Inport  Port=3
  Normal Pitch Coefficient : Inport  Port=4
  Planar Area : Inport  Port=5
  Normal Yaw Coefficient : Inport  Port=6
  Thrust : Inport  Port=7
  Dyn Presssure Yaw : Inport  Port=8
  Dynamic Pressure Pitch : Inport  Port=9
  Add : Sum  Inputs=+-
  Product : Product  Inputs=3
  Product1 : Product  Inputs=3
  Product2 : Product  Inputs=3
  Scope{,1..6} (7 alike) : Scope
  Axial Force : Outport  VectorParamsAs1DForOutWhenUnconnected=off
  Pitch Force : Outport  Port=2  VectorParamsAs1DForOutWhenUnconnected=off
  Yaw Force : Outport  Port=3  VectorParamsAs1DForOutWhenUnconnected=off
  wires:
  Cross Section/1 -> Product2/2, Product1/2, Product/2
  Product1/1 -> Pitch Force/1
  Product2/1 -> Scope5/1, Yaw Force/1
  Product/1 -> Scope1/1, Add/2
  Thrust/1 -> Add/1
  Axial Coefficient/1 -> Scope/1, Scope2/1, Product/1
  Dynamic Pressure Axial/1 -> Scope3/1, Product/3
  Add/1 -> Axial Force/1
  Normal Pitch Coefficient/1 -> Scope4/1, Product1/1
  Normal Yaw Coefficient/1 -> Product2/1
  Dyn Presssure Yaw/1 -> Scope6/1, Product2/3
  Dynamic Pressure Pitch/1 -> Product1/3

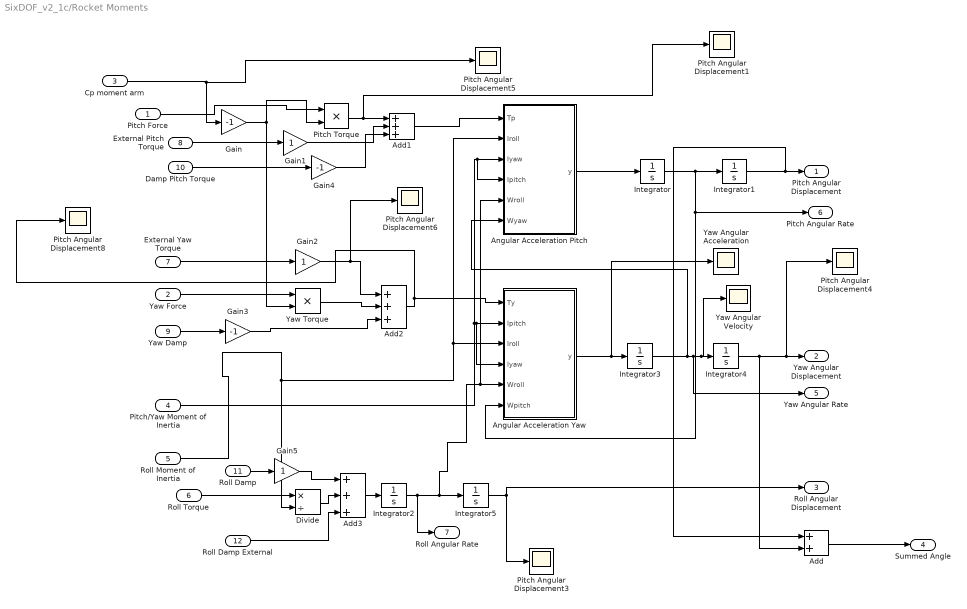
== system SixDOF_v2_1c/Rocket Moments ==
  Pitch Force : Inport
  Yaw Force : Inport  Port=2
  Cp moment arm : Inport  Port=3
  Pitch/Yaw Moment of Inertia : Inport  Port=4
  Roll Moment of Inertia : Inport  Port=5
  Roll Torque : Inport  Port=6
  External Yaw Torque : Inport  Port=7
  External Pitch Torque : Inport  Port=8
  Yaw Damp : Inport  Port=9
  Damp Pitch Torque : Inport  Port=10
  Roll Damp : Inport  Port=11
  Roll Damp External : Inport  Port=12
  Add : Sum
  Add1 : Sum  Inputs=+++
  Add2 : Sum  Inputs=+++
  Add3 : Sum  Inputs=+++
  Angular Acceleration Pitch : MATLAB Function  TreatAsAtomicUnit=on
  Angular Acceleration Yaw : MATLAB Function  TreatAsAtomicUnit=on
  Divide : Product  Inputs=*/
  Gain : Gain  Gain=-1
  Gain1 : Gain
  Gain2 : Gain
  Gain3 : Gain  Gain=-1
  Gain4 : Gain  Gain=-1
  Gain5 : Gain
  Integrator{,1..5} (6 alike) : Integrator
  Pitch Angular Displacement{1,3..6,8} (6 alike) : Scope
  Pitch Torque : Product
  Yaw Angular Acceleration : Scope
  Yaw Angular Velocity : Scope
  Yaw Torque : Product
  Pitch Angular Displacement : Outport  VectorParamsAs1DForOutWhenUnconnected=off
  Yaw Angular Displacement : Outport  Port=2  VectorParamsAs1DForOutWhenUnconnected=off
  Roll Angular Displacement : Outport  Port=3  VectorParamsAs1DForOutWhenUnconnected=off
  Summed Angle : Outport  Port=4  VectorParamsAs1DForOutWhenUnconnected=off
  Yaw Angular Rate : Outport  Port=5  VectorParamsAs1DForOutWhenUnconnected=off
  Pitch Angular Rate : Outport  Port=6  VectorParamsAs1DForOutWhenUnconnected=off
  Roll Angular Rate : Outport  Port=7  VectorParamsAs1DForOutWhenUnconnected=off
  wires:
  Integrator1/1 -> Add/1, Pitch Angular Displacement/1
  Integrator/1 -> Angular Acceleration Yaw/6(Wpitch), Pitch Angular Rate/1, Integrator1/1
  Add/1 -> Summed Angle/1
  Integrator2/1 -> Roll Angular Rate/1, Angular Acceleration Pitch/5(Wroll), Angular Acceleration Yaw/5(Wroll), Integrator5/1
  Integrator5/1 -> Roll Angular Displacement/1, Pitch Angular Displacement3/1
  Add1/1 -> Angular Acceleration Pitch/1(Tp)
  Pitch Torque/1 -> Pitch Angular Displacement1/1, Add1/1
  Yaw Torque/1 -> Add2/2
  Add2/1 -> Pitch Angular Displacement8/1, Angular Acceleration Yaw/1(Ty)
  Gain/1 -> Yaw Torque/2, Pitch Torque/2
  Cp moment arm/1 -> Pitch Angular Displacement5/1, Gain/1
  Pitch/Yaw Moment of Inertia/1 -> Angular Acceleration Pitch/4(Ipitch), Angular Acceleration Pitch/3(Iyaw), Angular Acceleration Yaw/4(Iyaw), Angular Acceleration Yaw/2(Ipitch)
  External Pitch Torque/1 -> Gain1/1
  Angular Acceleration Pitch/1(y) -> Integrator/1
  Pitch Force/1 -> Pitch Torque/1
  External Yaw Torque/1 -> Gain2/1
  Roll Moment of Inertia/1 -> Divide/2, Angular Acceleration Pitch/2(Iroll), Angular Acceleration Yaw/3(Iroll)
  Roll Torque/1 -> Divide/1
  Gain1/1 -> Add1/2
  Gain2/1 -> Pitch Angular Displacement6/1, Add2/1
  Gain3/1 -> Add2/3
  Yaw Damp/1 -> Gain3/1
  Angular Acceleration Yaw/1(y) -> Yaw Angular Acceleration/1, Integrator3/1
  Integrator4/1 -> Pitch Angular Displacement4/1, Yaw Angular Displacement/1, Add/2
  Integrator3/1 -> Yaw Angular Velocity/1, Integrator4/1, Yaw Angular Rate/1, Angular Acceleration Pitch/6(Wyaw)
  Yaw Force/1 -> Yaw Torque/1
  Damp Pitch Torque/1 -> Gain4/1
  Gain4/1 -> Add1/3
  Divide/1 -> Add3/2
  Roll Damp/1 -> Gain5/1
  Add3/1 -> Integrator2/1
  Roll Damp External/1 -> Add3/3
  Gain5/1 -> Add3/1

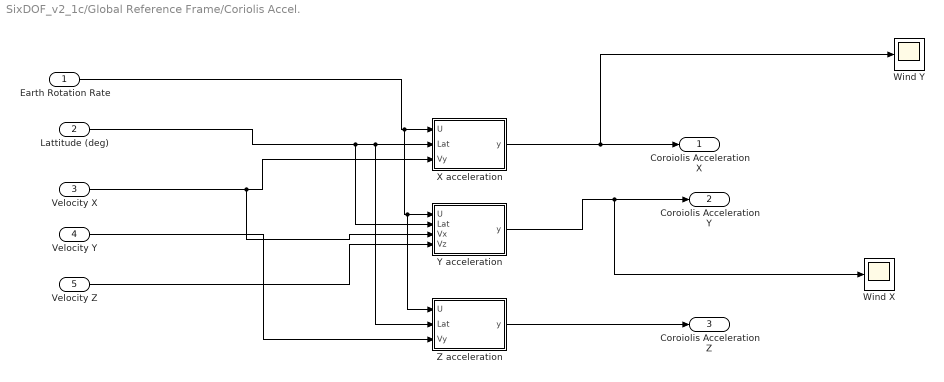
== system SixDOF_v2_1c/Global Reference Frame/Coriolis Accel. ==
  Earth Rotation Rate : Inport
  Lattitude (deg) : Inport  Port=2
  Velocity X : Inport  Port=3
  Velocity Y : Inport  Port=4
  Velocity Z : Inport  Port=5
  Wind X : Scope
  Wind Y : Scope
  X acceleration : MATLAB Function  TreatAsAtomicUnit=on
  Y acceleration : MATLAB Function  TreatAsAtomicUnit=on
  Z acceleration : MATLAB Function  TreatAsAtomicUnit=on
  Coroiolis Acceleration X : Outport  VectorParamsAs1DForOutWhenUnconnected=off
  Coroiolis Acceleration Y : Outport  Port=2  VectorParamsAs1DForOutWhenUnconnected=off
  Coroiolis Acceleration Z : Outport  Port=3  VectorParamsAs1DForOutWhenUnconnected=off
  wires:
  Earth Rotation Rate/1 -> Z acceleration/1(U), Y acceleration/1(U), X acceleration/1(U)
  Lattitude (deg)/1 -> Y acceleration/2(Lat), Z acceleration/2(Lat), X acceleration/2(Lat)
  Velocity X/1 -> Y acceleration/3(Vx), X acceleration/3(Vy)
  Velocity Y/1 -> Z acceleration/3(Vy)
  Velocity Z/1 -> Y acceleration/4(Vz)
  X acceleration/1(y) -> Wind Y/1, Coroiolis Acceleration X/1
  Y acceleration/1(y) -> Wind X/1, Coroiolis Acceleration Y/1
  Z acceleration/1(y) -> Coroiolis Acceleration Z/1

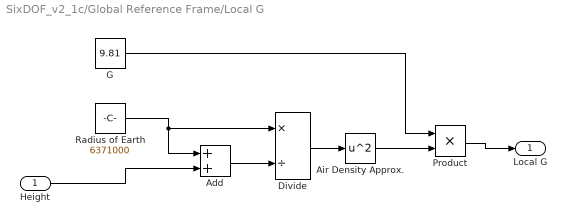
== system SixDOF_v2_1c/Global Reference Frame/Local G ==
  Height : Inport
  Add : Sum
  Air Density Approx. : Math  Operator=square  OutMin=0  OutMax=10000  SaturateOnIntegerOverflow=on
  Divide : Product  Inputs=*/
  G : Constant  Value=9.81
  Product : Product
  Radius of Earth : Constant  Value=6371000
  Local G : Outport  VectorParamsAs1DForOutWhenUnconnected=off
  wires:
  Radius of Earth/1 -> Divide/1, Add/1
  Height/1 -> Add/2
  Add/1 -> Divide/2
  Divide/1 -> Air Density Approx./1
  Air Density Approx./1 -> Product/2
  Product/1 -> Local G/1
  G/1 -> Product/1

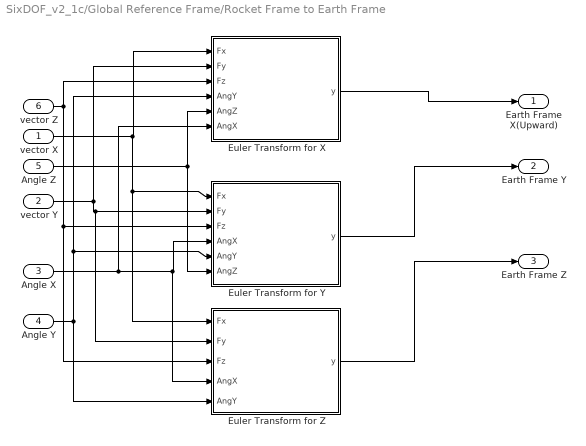
== system SixDOF_v2_1c/Global Reference Frame/Rocket Frame to Earth Frame ==
  vector X : Inport
  vector Y : Inport  Port=2
  Angle X : Inport  Port=3
  Angle Y : Inport  Port=4
  Angle Z : Inport  Port=5
  vector Z : Inport  Port=6
  Euler Transform for X : MATLAB Function  TreatAsAtomicUnit=on
  Euler Transform for Y : MATLAB Function  TreatAsAtomicUnit=on
  Euler Transform for Z : MATLAB Function  TreatAsAtomicUnit=on
  Earth Frame X(Upward) : Outport  VectorParamsAs1DForOutWhenUnconnected=off
  Earth Frame Y : Outport  Port=2  VectorParamsAs1DForOutWhenUnconnected=off
  Earth Frame Z : Outport  Port=3  VectorParamsAs1DForOutWhenUnconnected=off
  wires:
  vector X/1 -> Euler Transform for Z/1(Fx), Euler Transform for Y/1(Fx), Euler Transform for X/1(Fx)
  vector Y/1 -> Euler Transform for X/2(Fy), Euler Transform for Z/2(Fy), Euler Transform for Y/2(Fy)
  Angle X/1 -> Euler Transform for X/6(AngX), Euler Transform for Z/4(AngX), Euler Transform for Y/4(AngX)
  Angle Y/1 -> Euler Transform for Y/5(AngY), Euler Transform for X/4(AngY), Euler Transform for Z/5(AngY)
  Angle Z/1 -> Euler Transform for Y/6(AngZ), Euler Transform for X/5(AngZ)
  Euler Transform for X/1(y) -> Earth Frame X(Upward)/1
  Euler Transform for Y/1(y) -> Earth Frame Y/1
  Euler Transform for Z/1(y) -> Earth Frame Z/1
  vector Z/1 -> Euler Transform for Z/3(Fz), Euler Transform for Y/3(Fz), Euler Transform for X/3(Fz)

== matlab function SixDOF_v2_1c/Rocket Moments/Angular Acceleration Yaw ==
  data: Ty input; Ipitch input; y output; Iroll input; Iyaw input; Wroll input; Wpitch input
function y = fcn(Ty, Ipitch, Iroll, Iyaw, Wroll,Wpitch)

y = (Ty - (Ipitch - Iroll)*Wroll*Wpitch)/Iyaw;

== matlab function SixDOF_v2_1c/Rocket Moments/Angular Acceleration Pitch ==
  data: Tp input; y output; Iroll input; Iyaw input; Ipitch input; Wroll input; Wyaw input
function y = fcn(Tp, Iroll, Iyaw, Ipitch, Wroll,Wyaw)

y = (Tp - (Iroll - Iyaw)*Wroll*Wyaw)/Ipitch;

== matlab function SixDOF_v2_1c/Global Reference Frame/MATLAB Function ==
  data: u input; y output; v input; z input
function y = fcn(u, v, z)

y = (u^2 + v^2 + z^2)^0.5;

== matlab function SixDOF_v2_1c/Rocket Aerodynamic Variables/Dynam Pressure ==
  data: rho input; y output; V input
function y = fcn(rho, V)

y = 0.5*rho*V^2;

== matlab function SixDOF_v2_1c/Rocket Dynamic Variables /MATLAB Function1 ==
  data: Po input; y output; Tb input; t input
function y = fcn(Po, Tb, t)
%#codegen

y = -(Po/Tb)*t+Po;

== matlab function SixDOF_v2_1c/Rocket Dynamic Variables /MATLAB Function2 ==
  data: CG_I input; CG_F input; y output; Tb input; t input
function y = fcn(CG_I, CG_F, Tb, t)
%#codegen

y = -((-CG_F+CG_I)/Tb)*t+CG_I;

== matlab function SixDOF_v2_1c/Atmospheric Var./MATLAB Function ==
  data: T input; y output
function y = fcn(T)

y = (1.4*8.314*T/0.02895)^0.5;

== matlab function SixDOF_v2_1c/Atomic Subsystem/MATLAB Function ==
  data: T input; u input; y output; h input; launchrail input
function y = fcn(T, u, h, launchrail)

if h > launchrail
y = T*sin(u);
else
    y = 0;
end

== matlab function SixDOF_v2_1c/Atomic Subsystem/MATLAB Function1 ==
  data: T input; u input; y output; h input; launchrail input
function y = fcn(T, u, h, launchrail)

if h > launchrail
y = T*sin(u);
else
    y = 0;
end

== matlab function SixDOF_v2_1c/Atomic Subsystem/MATLAB Function2 ==
  data: T input; u input; y output; h input; launchrail input
function y = fcn(T, u, h, launchrail)

if h > launchrail
y = T*u;
else
    y = 0;
end

== matlab function SixDOF_v2_1c/Rocket Aerodynamic Variables/Dynam Pressure1 ==
  data: a input; rho input; y output; V input
function y = fcn(a, rho, V)

y = sin(a)*0.5*rho*V^2;

== matlab function SixDOF_v2_1c/Rocket Aerodynamic Variables/Dynam Pressure2 ==
  data: a input; rho input; y output; V input
function y = fcn(a, rho, V)

y = sin(a)*0.5*rho*V^2;

== matlab function SixDOF_v2_1c/Atomic Subsystem1/MATLAB Function ==
  data: w input; y output; d input; Cd input; a input; b input; Dyn input
function y = fcn(w, d, Cd, a, b, Dyn)

y = abs(w)/((w+(w==0)*eps))*w^2*d*Cd*(b^3 - a^3)/3*Dyn;

== matlab function SixDOF_v2_1c/Atomic Subsystem1/MATLAB Function1 ==
  data: w input; y output; d input; Cd input; a input; b input; Dyn input
function y = fcn(w, d, Cd, a, b, Dyn)

y = abs(w)/((w+(w==0)*eps))*w^2*d*Cd*(b^3 - a^3)/3*Dyn;

== matlab function SixDOF_v2_1c/Atomic Subsystem1/MATLAB Function2 ==
  data: w input; y output; r input; Area input; Dyn input
function y = fcn(w, r, Area, Dyn)

y = abs(w)/((w+(w==0)*eps))*w^2*r^3*Area*Dyn*2;

== matlab function SixDOF_v2_1c/Atomic Subsystem1/MATLAB Function3 ==
  data: w input; y output; d input; Cd input; a input; b input; Dyn input
function y = fcn(w, d, Cd, a, b, Dyn)

y = abs(w)/((w+(w==0)*eps))*w^2*d*Cd*(b^3 - a^3)/3*Dyn;

== matlab function SixDOF_v2_1c/MATLAB Function ==
  data: M input; D input; y output; L input
function y = fcn(M, D, L)

y = 1/4*M*(D/2)^2+1/12*M*L^2;

== matlab function SixDOF_v2_1c/MATLAB Function1 ==
  data: M input; D input; y output
function y = fcn(M, D)

y = 1/2*M*(D/2)^2;

== matlab function SixDOF_v2_1c/Atomic Subsystem1/MATLAB Function4 ==
  data: w input; y output; d input; Cd input; a input; b input; Dyn input
function y = fcn(w, d, Cd, a, b, Dyn)

y = abs(w)/((w+(w==0)*eps))*w^2*d*Cd*(b^3 - a^3)/3*Dyn;

== matlab function SixDOF_v2_1c/Atomic Subsystem1/MATLAB Function5 ==
  data: w input; y output; r input; Area input; Dyn input
function y = fcn(w, r, Area, Dyn)

y = abs(w)/((w+(w==0)*eps))*w^2*r^3*Area*Dyn*2;

== matlab function SixDOF_v2_1c/Global Reference Frame/Coriolis Accel./X acceleration ==
  data: U input; y output; Lat input; Vy input
function y = fcn(U, Lat, Vy)

y = 2*U*sind(Lat)*Vy;

== matlab function SixDOF_v2_1c/Global Reference Frame/Coriolis Accel./Y acceleration ==
  data: U input; y output; Lat input; Vx input; Vz input
function y = fcn(U, Lat, Vx, Vz)

y = -2*U*sind(Lat)*Vx -2*U*cosd(Lat)*Vz;

== matlab function SixDOF_v2_1c/Global Reference Frame/Coriolis Accel./Z acceleration ==
  data: U input; y output; Lat input; Vy input
function y = fcn(U, Lat, Vy)

y = -2*U*cosd(Lat)*Vy;

== matlab function SixDOF_v2_1c/MATLAB Function2 ==
  data: alpha input; magAngle1 input; magAngle2 input; y output; rho input; V input; FinBaseLgth input; FinTipLgth input; FinSpan input; RocketDiameter input
function y = fcn(alpha,magAngle1,magAngle2,rho,V,FinBaseLgth,FinTipLgth,FinSpan,RocketDiameter)
b = FinBaseLgth - FinTipLgth;
a = FinTipLgth;
c = FinSpan;
r = RocketDiameter/2;
Q = 1/2*rho*V*abs(V);
Cd = 0.45;
Ta = Cd*Q*(b/2*(r+c)^3 - b*(r+c)^3/3 - b/2*r^2*(c+r)/2+b*r^3/3)/c;
Tb = Cd*Q*a*(r+c)^3/2-r*(r+c)^2/2;
y = 2*sin(alpha+magAngle1)*(Ta+Tb)+2*sin(alpha+magAngle2)*(Ta+Tb);

== matlab function SixDOF_v2_1c/Atomic Subsystem1/Roll Damp1 ==
  data: Cm_d input; Q input; FinArea input; w input; y output
function y = fcn(Cm_d,Q,FinArea,w)

y = 4*w*FinArea*Q*Cm_d;

== matlab function SixDOF_v2_1c/Global Reference Frame/Rocket Frame to Earth Frame/Euler Transform for X ==
  data: Fx input; y output; Fy input; Fz input; AngY input; AngZ input; AngX input
function y = fcn(Fx, Fy, Fz, AngY, AngZ, AngX)
%#codegen

y = Fx*(cos(AngY)*cos(AngZ)) + Fy*(sin(AngX)*sin(AngY)*cos(AngZ)-cos(AngX)*sin(AngZ)) + Fz*(sin(AngX)*sin(AngZ)+cos(AngX)*sin(AngY)*cos(AngZ));

== matlab function SixDOF_v2_1c/Global Reference Frame/Rocket Frame to Earth Frame/Euler Transform for Y ==
  data: Fx input; y output; Fy input; Fz input; AngX input; AngY input; AngZ input
function y = fcn(Fx, Fy, Fz, AngX, AngY, AngZ)
%#codegen

y = Fx*(cos(AngY))*sin(AngZ)+Fy*(cos(AngX)*cos(AngZ)+sin(AngX)*sin(AngY)*sin(AngZ)) + Fz*(cos(AngX)*sin(AngY)*sin(AngZ)-sin(AngX)*cos(AngZ));

== matlab function SixDOF_v2_1c/Global Reference Frame/Rocket Frame to Earth Frame/Euler Transform for Z ==
  data: Fx input; y output; Fy input; Fz input; AngX input; AngY input
function y = fcn(Fx, Fy, Fz, AngX, AngY)
%#codegen

y = -Fx*sin(AngY) + Fy*(sin(AngX)*cos(AngY)) + Fz*(cos(AngX)*sin(AngY));

== matlab function SixDOF_v2_1c/MATLAB Function3 ==
  data: y output; FinBaseLgth input; FinTipLgth input; FinSpan input
function y = fcn(FinBaseLgth,FinTipLgth,FinSpan)
y = (FinBaseLgth-FinTipLgth)*FinSpan/2+FinSpan*FinTipLgth;

== matlab function SixDOF_v2_1c/Atomic Subsystem1/Roll Damp ==
  data: Cd input; N input; rollrate input; a input; b input; c input; y output; r input
function y = fcn(Cd,N,rollrate,a,b,c,r)
Q = Cd*N*rollrate*abs(rollrate);
Ta = 4*Q*(b/20*(r+c)^5 - b/4*r^5*(r+c)+r^5/5);
Tb = 4*Q*a*((r+c)^4/4 - r*(r+c)^3/3 - r^4/4 + r^4/3);
y = Ta+Tb;
